simulink model "SAR"  (R2016a)
settings: Solver=VariableStepAuto  StartTime=0.0  StopTime=.1  RelTol=1e-3
libraries: dspsigops x3, simulink x1
settings Model: Creator=ucagu  LastModifiedBy=ucagu

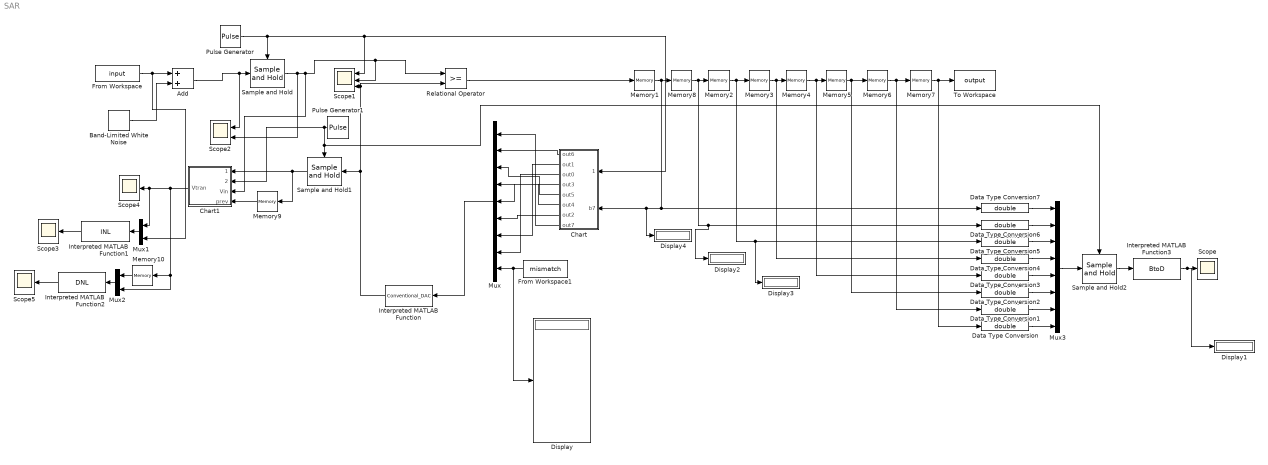
== system SAR ==
  Add : Sum
  Band-Limited White Noise : simulink/Sources/Band-Limited White Noise  Cov=0  Ts=1e-4  seed=[23341]
  Chart : Stateflow chart  TreatAsAtomicUnit=on
  Chart1 : Stateflow chart  TreatAsAtomicUnit=on
  Data Type Conversion{,1..7} (8 alike) : DataTypeConversion  OutDataTypeStr=double
  Display{,1..4} (5 alike) : Display
  From Workspace : FromWorkspace  VariableName=input  SampleTime=1e-5
  From Workspace1 : FromWorkspace  VariableName=mismatch  SampleTime=0
  Interpreted MATLAB Function : MATLABFcn  MATLABFcn=Conventional_DAC
  Interpreted MATLAB Function1 : MATLABFcn  MATLABFcn=INL
  Interpreted MATLAB Function2 : MATLABFcn  MATLABFcn=DNL
  Interpreted MATLAB Function3 : MATLABFcn  MATLABFcn=BtoD
  Memory{1..10} (10 alike) : Memory  InheritSampleTime=on  LinearizeAsDelay=on
  Mux : Mux  Inputs=9
  Mux1 : Mux  Inputs=2
  Mux2 : Mux  Inputs=2
  Mux3 : Mux  Inputs=8
  Pulse Generator : DiscretePulseGenerator  PulseType=Time based  Period=.002  PulseWidth=50
  Pulse Generator1 : DiscretePulseGenerator  PulseType=Time based  Period=.002  PulseWidth=50  PhaseDelay=.0015
  Relational Operator : RelationalOperator  OutDataTypeStr=boolean
  Sample and Hold : dspsigops/Sample and Hold  trig=Rising edge  initCond=0  latchinput=off
  Sample and Hold1 : dspsigops/Sample and Hold  trig=Rising edge  initCond=0  latchinput=off
  Sample and Hold2 : dspsigops/Sample and Hold  trig=Rising edge  initCond=0  latchinput=off
  Scope{,3..5} (4 alike) : Scope
  Scope1 : Scope  NumInputPorts=3
  Scope2 : Scope  NumInputPorts=2
  To Workspace : ToWorkspace  VariableName=output  SaveFormat=Timeseries  SampleTime=-1
  wires:
  Pulse Generator/1 -> Scope1/1, Chart/1(enable), Sample and Hold/Trigger
  Relational Operator/1 -> Memory1/1
  Memory1/1 -> Memory8/1, Data Type Conversion7/1, Display4/1, Chart/2(b7)
  Memory2/1 -> Display3/1, Data Type Conversion5/1, Memory3/1
  Memory8/1 -> Display2/1, Data Type Conversion6/1, Memory2/1
  Memory3/1 -> Data Type Conversion4/1, Memory4/1
  Memory4/1 -> Data Type Conversion3/1, Memory5/1
  Memory6/1 -> Data Type Conversion1/1, Memory7/1
  Memory5/1 -> Data Type Conversion2/1, Memory6/1
  Memory7/1 -> Data Type Conversion/1, To Workspace/1
  Chart/3(out0) -> Mux/8
  Chart/2(out1) -> Mux/7
  Chart/7(out2) -> Mux/6
  Chart/4(out3) -> Mux/5
  Chart/6(out4) -> Mux/4
  Chart/5(out5) -> Mux/3
  Chart/1(out6) -> Mux/2
  Chart/8(out7) -> Mux/1
  Sample and Hold/1 -> Scope2/2, Chart1/3(Vin), Scope1/2, Relational Operator/1
  From Workspace/1 -> Mux1/2, Add/1
  Add/1 -> Scope2/1, Sample and Hold/1
  Band-Limited White Noise/1 -> Add/2
  Mux/1 -> Interpreted MATLAB Function/1
  From Workspace1/1 -> Display/1, Mux/9
  Interpreted MATLAB Function/1 -> Sample and Hold1/1, Scope1/3, Relational Operator/2
  Pulse Generator1/1 -> Chart1/2(enable), Sample and Hold2/Trigger, Sample and Hold1/Trigger
  Mux1/1 -> Interpreted MATLAB Function1/1
  Interpreted MATLAB Function1/1 -> Scope3/1
  Sample and Hold1/1 -> Chart1/1(current), Memory9/1
  Memory9/1 -> Chart1/4(prev)
  Chart1/1(Vtran) -> Mux2/2, Memory10/1, Mux1/1, Scope4/1
  Mux2/1 -> Interpreted MATLAB Function2/1
  Interpreted MATLAB Function2/1 -> Scope5/1
  Memory10/1 -> Mux2/1
  Mux3/1 -> Sample and Hold2/1
  Data Type Conversion/1 -> Mux3/8
  Data Type Conversion1/1 -> Mux3/7
  Data Type Conversion2/1 -> Mux3/6
  Data Type Conversion5/1 -> Mux3/3
  Data Type Conversion6/1 -> Mux3/2
  Data Type Conversion7/1 -> Mux3/1
  Sample and Hold2/1 -> Interpreted MATLAB Function3/1
  Data Type Conversion3/1 -> Mux3/5
  Data Type Conversion4/1 -> Mux3/4
  Interpreted MATLAB Function3/1 -> Display1/1, Scope/1

== stateflow chart SAR/Chart1 ==
  settings: updateMethod=DISCRETE  sampleTime=0.0001
  state wait
  state tran
    entry: Vtran = Vin;
  (default) -> wait
  wait -> tran : [current > prev & enable == 1]
  tran -> wait : [enable == 0]
  data: current input; enable input; Vin input; prev input; Vtran output

== stateflow chart SAR/Chart ==
  settings: updateMethod=DISCRETE  sampleTime=5e-5
  state B6
    entry: out6 = 1;
  state B5
    entry: out5 = 1;
  state B4
    entry: out4 = 1;
  state B3
    entry: out3 = 1;
  state B2
    entry: out2 = 1;
  state B1
    entry: out1 = 1;
  state B0
    entry: out0 = 1;
  state B8
    entry: out7 = 1;
    entry: out6 = 0;
    entry: out5 = 0;
    entry: out4 = 0;
    entry: out3 = 0;
    entry: out2 = 0;
    entry: out1 = 0;
    entry: out0 = 0;
  state B10
    entry: out6 = 1;
    entry: out7 = 0;
  state B12
    entry: out5 = 1;
    entry: out6 = 0;
  state B15
    entry: out4 = 1;
    entry: out5 = 0;
  state B14
    entry: out3 = 1;
    entry: out4 = 0;
  state B13
    entry: out2 = 1;
    entry: out3 = 0;
  state B9
    entry: out1 = 1;
    entry: out2 = 0;
  state B01
    entry: out0 = 1;
    entry: out1 = 0;
  B0 -> B8 : [enable==1]
  (default) -> B8
  B8 -> B6 [order 1] : [b7==1 & enable == 0]
  B6 -> B5 [order 1] : [b7 == 1]
  B5 -> B4 [order 1] : [b7 == 1]
  B4 -> B3 [order 1] : [b7 == 1]
  B3 -> B2 [order 1] : [b7 == 1]
  B2 -> B1 [order 1] : [b7 == 1]
  B1 -> B0 [order 1] : [b7 == 1]
  B9 -> B0 [order 2] : [b7 == 1]
  B3 -> B13 [order 2] : [b7 == 0]
  B14 -> B2 [order 2] : [b7 == 1]
  B6 -> B12 [order 2] : [b7 == 0]
  B13 -> B1 [order 2] : [b7 ==1]
  B4 -> B14 [order 2] : [b7 == 0]
  B2 -> B9 [order 2] : [b7 == 0]
  B12 -> B4 [order 2] : [b7 == 1]
  B5 -> B15 [order 2] : [b7 == 0]
  B10 -> B5 [order 2] : [b7 == 1]
  B15 -> B3 [order 2] : [b7 == 1]
  B1 -> B01 [order 2] : [b7 == 0]
  B8 -> B10 [order 2] : [b7 == 0 & enable == 0]
  B10 -> B12 [order 1] : [b7 == 0]
  B12 -> B15 [order 1] : [b7 == 0]
  B15 -> B14 [order 1] : [b7 == 0]
  B14 -> B13 [order 1] : [b7 == 0]
  B13 -> B9 [order 1] : [b7 == 0]
  B9 -> B01 [order 1] : [b7 == 0]
  B01 -> B8 : [enable == 1]
  data: enable input; b7 input; out6 output; out1 output; out0 output; out3 output; out5 output; out4 output; out2 output; out7 output
